simulink model "lab1"  (R2020b)
settings: Solver=VariableStepAuto  StartTime=0.0  StopTime=10.0  RelTol=1e-3
libraries: simulink x1
settings Model: Creator=Олег  LastModifiedBy=Олег

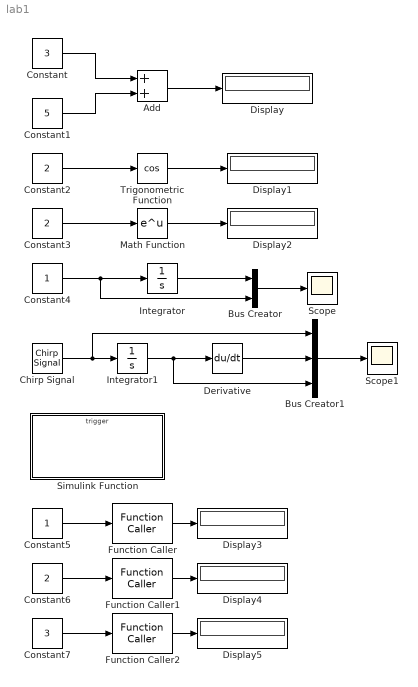
== system lab1 ==
  Add : Sum
  Bus Creator : BusCreator  Inputs=2
  Bus Creator1 : BusCreator  Inputs=3
  Chirp Signal : simulink/Sources/Chirp Signal  f1=0.1  T=100  f2=1
  Constant : Constant  Value=3
  Constant1 : Constant  Value=5
  Constant2 : Constant  Value=2
  Constant3 : Constant  Value=2
  Constant4 : Constant
  Constant5 : Constant
  Constant6 : Constant  Value=2
  Constant7 : Constant  Value=3
  Derivative : Derivative
  Display{,1..5} (6 alike) : Display
  Function Caller : FunctionCaller  FunctionPrototype=y = f(x)  InputArgumentSpecifications=<Enter example>  OutputArgumentSpecifications=<Enter example>
  Function Caller1 : FunctionCaller  FunctionPrototype=y = f(x)  InputArgumentSpecifications=<Enter example>  OutputArgumentSpecifications=<Enter example>
  Function Caller2 : FunctionCaller  FunctionPrototype=y = f(x)  InputArgumentSpecifications=<Enter example>  OutputArgumentSpecifications=<Enter example>
  Integrator : Integrator
  Integrator1 : Integrator
  Math Function : Math  SaturateOnIntegerOverflow=on
  Scope : Scope
  Scope1 : Scope
  Simulink Function : Subsystem  TreatAsAtomicUnit=on
  Trigonometric Function : Trigonometry  Operator=cos
  wires:
  Constant1/1 -> Add/2
  Constant/1 -> Add/1
  Add/1 -> Display/1
  Constant2/1 -> Trigonometric Function/1
  Trigonometric Function/1 -> Display1/1
  Constant3/1 -> Math Function/1
  Math Function/1 -> Display2/1
  Bus Creator/1 -> Scope/1
  Integrator/1 -> Bus Creator/1
  Constant4/1 -> Bus Creator/2, Integrator/1
  Bus Creator1/1 -> Scope1/1
  Derivative/1 -> Bus Creator1/2
  Integrator1/1 -> Bus Creator1/3, Derivative/1
  Chirp Signal/1 -> Bus Creator1/1, Integrator1/1
  Constant5/1 -> Function Caller/1
  Function Caller/1 -> Display3/1
  Constant6/1 -> Function Caller1/1
  Function Caller1/1 -> Display4/1
  Constant7/1 -> Function Caller2/1
  Function Caller2/1 -> Display5/1

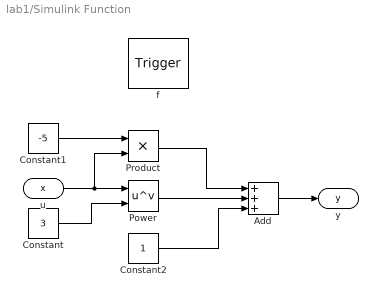
== system lab1/Simulink Function ==
  f : TriggerPort  TriggerType=function-call  IsSimulinkFunction=on  FunctionName=f  FunctionVisibility=scoped  VariantControl=(inherit)
  Add : Sum  Inputs=+++
  Constant : Constant  Value=3
  Constant1 : Constant  Value=-5
  Constant2 : Constant
  Power : Math  Operator=pow  SaturateOnIntegerOverflow=on
  Product : Product
  u : ArgIn  DisableCoverage=on  ArgumentName=x
  y : ArgOut  DisableCoverage=on  ArgumentName=y
  wires:
  u/1 -> Product/2, Power/1
  Constant/1 -> Power/2
  Power/1 -> Add/2
  Constant1/1 -> Product/1
  Product/1 -> Add/1
  Constant2/1 -> Add/3
  Add/1 -> y/1
